simulink model "TASK_2"  (R2018b)
settings: Solver=VariableStepAuto  StartTime=0.0  StopTime=10  RelTol=1e-3
libraries: simulink x4
settings Model: Creator=Федор  LastModifiedBy=Федор

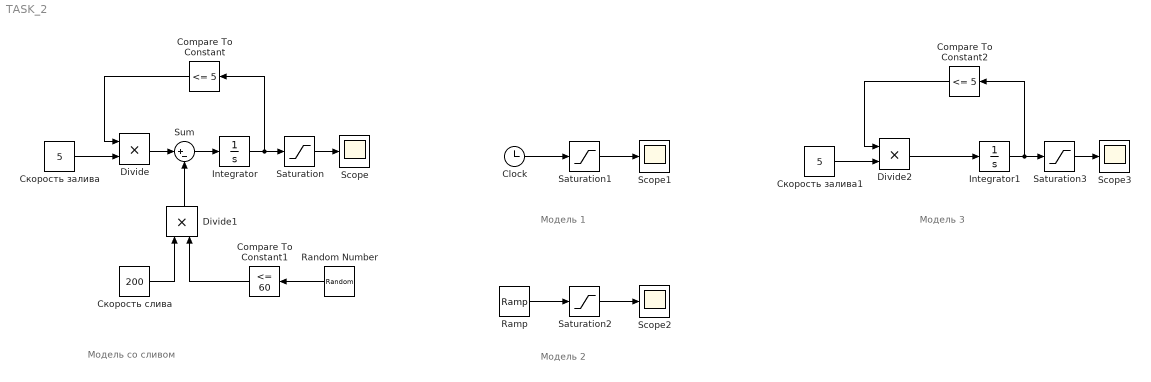
== system TASK_2 ==
  note: Модель со сливом
  note: Модель 1
  note: Модель 2
  note: Модель 3
  Clock : Clock
  Compare To Constant : simulink/Logic and Bit Operations/Compare To Constant  relop=<=  const=5  OutDataTypeStr=boolean
  Compare To Constant1 : simulink/Logic and Bit Operations/Compare To Constant  relop=<=  const=60  OutDataTypeStr=uint8  ZeroCross=off
  Compare To Constant2 : simulink/Logic and Bit Operations/Compare To Constant  relop=<=  const=5  OutDataTypeStr=boolean
  Divide : Product  Inputs=**
  Divide1 : Product  Inputs=**
  Divide2 : Product  Inputs=**
  Integrator : Integrator
  Integrator1 : Integrator
  Ramp : simulink/Sources/Ramp  slope=1  start=0  InitialOutput=0
  Random Number : RandomNumber  Mean=80  Variance=80  Seed=0.1  SampleTime=0.1
  Saturation : Saturate  UpperLimit=inf  LowerLimit=0
  Saturation1 : Saturate  UpperLimit=5  LowerLimit=0
  Saturation2 : Saturate  UpperLimit=5  LowerLimit=0
  Saturation3 : Saturate  UpperLimit=inf  LowerLimit=0
  Scope{,1..3} (4 alike) : Scope
  Sum : Sum  Inputs=|+-
  Скорость залива : Constant  Value=5
  Скорость залива1 : Constant  Value=5
  Скорость слива : Constant  Value=200
  wires:
  Integrator/1 -> Saturation/1, Compare To Constant/1
  Скорость залива/1 -> Divide/2
  Compare To Constant/1 -> Divide/1
  Divide/1 -> Sum/1
  Sum/1 -> Integrator/1
  Divide1/1 -> Sum/2
  Скорость слива/1 -> Divide1/1
  Random Number/1 -> Compare To Constant1/1
  Compare To Constant1/1 -> Divide1/2
  Saturation/1 -> Scope/1
  Clock/1 -> Saturation1/1
  Saturation1/1 -> Scope1/1
  Ramp/1 -> Saturation2/1
  Saturation2/1 -> Scope2/1
  Integrator1/1 -> Saturation3/1, Compare To Constant2/1
  Compare To Constant2/1 -> Divide2/1
  Saturation3/1 -> Scope3/1
  Скорость залива1/1 -> Divide2/2
  Divide2/1 -> Integrator1/1
